simulink model "modelo_pink_noise"  (R2020a)
settings: Solver=ode15s  StartTime=0.0  StopTime=10  FixedStep=1/fs  MaxStep=1/(fs)  RelTol=1e-6
undefined symbols (not defined in the file): A, A_reduc, Amp, B, B_reduc, ba, Bdlol, C_reduc, Cc, D, den_anti, den_mems, dfilt, DiscIntNeverNeededParam, f0, fs, g, K_motor_virtual, ksi, ksia, L, Li, Lobs, n_adc, NSD_mems, num_anti, num_mems, obs_i_den, obs_i_num, obs_x2_den, obs_x2_num, R, R_control, sens_mems, v0, V_max, Vcc, Vmax_ADC, Vmin_ADC, x0
libraries: simulink x1, dspstat3 x1, dsparch4 x1, simulink_extras x1
settings Model: Creator=Noxi-PC  LastModifiedBy=Noxi-PC
settings SolverCC: ZeroCrossAlgorithm=Adaptive
settings DebuggingCC: IgnoredZcDiagnostic=none

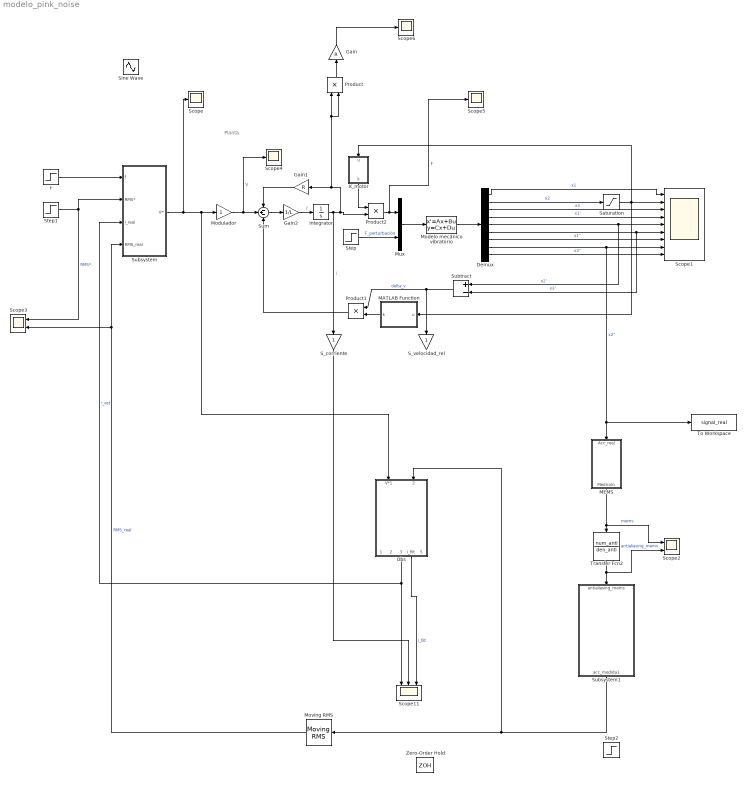
== system modelo_pink_noise ==
  note: Planta
  Demux : Demux  Outputs=9
  Gain : Gain  Gain=R
  Gain1 : Gain  Gain=R
  Gain2 : Gain  Gain=1/L
  Integrator : Integrator
  K_motor : MATLAB Function  TreatAsAtomicUnit=on
  MATLAB Function : MATLAB Function  TreatAsAtomicUnit=on
  MEMS : Subsystem
  Modelo mecánico vibratorio : StateSpace  A=A  B=B  C=Cc  D=D  InitialCondition=[x0,v0]
  Modulador : Gain
  Moving RMS : dspstat3/Moving RMS  Method=Sliding window  ForgettingFactorPort=off  SpecifyWindowLength=on  WindowLength=Ventana  ForgettingFactor=0.99  SimulateUsing=Interpreted execution
      settings: SourceProductBaseCode=DS
  Mux : Mux  Inputs=2
  Obs : Subsystem
  Product : Product
  Product1 : Product
  Product2 : Product
  S_corriente : Gain
  S_velocidad_rel : Gain
  Saturation : Saturate  UpperLimit=12.7e-3  LowerLimit=-12.7e-3
  Scope{,4..6} (4 alike) : Scope
  Scope1 : Scope  NumInputPorts=9
  Scope11 : Scope  NumInputPorts=3
  Scope2 : Scope  NumInputPorts=2
  Scope3 : Scope  NumInputPorts=2
  Sine Wave : Sin  Amplitude=5  Frequency=2*pi*f0  SampleTime=0
  Step : Step  After=0  SampleTime=0
  Step1 : Step  Time=0  After=Amp/sqrt(2)  SampleTime=0
  Step2 : Step  SampleTime=0
  Subsystem : Subsystem
  Subsystem1 : Subsystem
  Subtract : Sum  Inputs=+-
  Sum : Sum  Inputs=-+-
  To Workspace : ToWorkspace  VariableName=signal_real  SaveFormat=Structure With Time  SampleTime=-1
  Transfer Fcn2 : TransferFcn  Numerator=num_anti  Denominator=den_anti
  Zero-Order Hold : ZeroOrderHold  SampleTime=1/fs
  f : Step  Time=0  After=f0  SampleTime=0
  wires:
  Modelo mecánico vibratorio/1 -> Demux/1
  Demux/1 -> Scope1/1  "x1"
  Demux/2 -> Saturation/1  "x2"
  Demux/3 -> Scope1/3  "x3"
  Demux/4 -> Scope1/4  "x1'"
  Demux/5 -> Scope1/5, Subtract/1  "x2'"
  Demux/6 -> Scope1/6, Subtract/2  "x3'"
  Demux/7 -> Scope1/7  "x1''"
  Demux/8 -> To Workspace/1, MEMS/1(Acc_real), Scope1/8  "x2''"
  Demux/9 -> Scope1/9  "x3''"
  Mux/1 -> Modelo mecánico vibratorio/1
  Sum/1 -> Gain2/1
  Integrator/1 -> S_corriente/1, Product2/2, Gain1/1, Product/2, Product/1  "i"
  Gain1/1 -> Sum/1
  Gain2/1 -> Integrator/1  "i'"
  Step/1 -> Mux/2  "F_perturbación"
  Product1/1 -> Sum/3
  Subtract/1 -> Product1/1, S_velocidad_rel/1  "delta_v"
  Modulador/1 -> Scope4/1, Sum/2  "V"
  Saturation/1 -> K_motor/1(u), MATLAB Function/1(u), Scope1/2
  Product2/1 -> Scope5/1, Mux/1  "F"
  K_motor/1(k) -> Product2/1
  MATLAB Function/1(k) -> Product1/2
  f/1 -> Subsystem/1(f)
  Step1/1 -> Subsystem/2(RMS*), Scope3/1  "RMS*"
  Subsystem/1(V*') -> Scope/1, Obs/1(V*1), Modulador/1
  MEMS/1(Medición) -> Scope2/1, Transfer Fcn2/1  "mems"
  Obs/3(i_est) -> Subsystem/3(i_real), Scope11/1  "i_est"
  Obs/4(i_filt) -> Scope11/3  "i_filt"
  Moving RMS/1 -> Subsystem/4(RMS_real), Scope3/2  "RMS_real"
  Transfer Fcn2/1 -> Scope2/2, Subsystem1/1(antialiasing_mems)  "antialiasing_mems"
  S_corriente/1 -> Scope11/2
  Subsystem1/1(acc_medida1) -> Obs/2(acc_medida1), Moving RMS/1
  Product/1 -> Gain/1
  Gain/1 -> Scope6/1

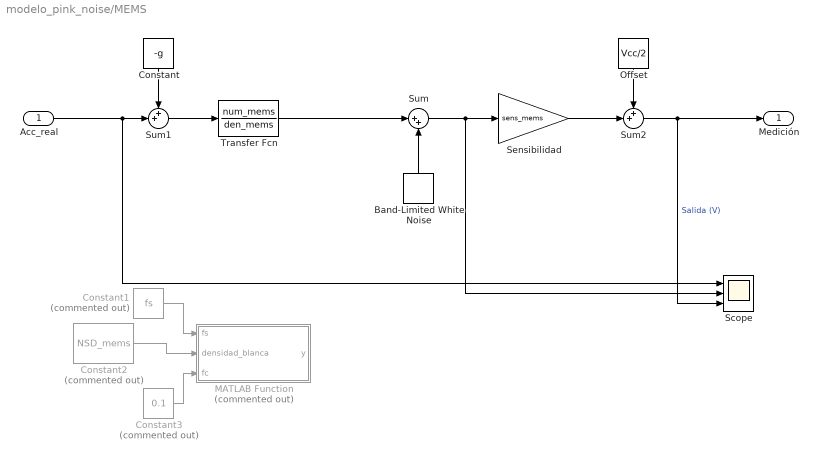
== system modelo_pink_noise/MEMS ==
  Acc_real : Inport
  Band-Limited White Noise : simulink/Sources/Band-Limited White Noise  Cov=NoisePower_mems  Ts=1/fs  seed=[23341]
  Constant : Constant  Value=-g
  Constant1 : Constant  Commented=on  Value=fs
  Constant2 : Constant  Commented=on  Value=NSD_mems
  Constant3 : Constant  Commented=on  Value=0.1
  MATLAB Function : MATLAB Function  Commented=on  TreatAsAtomicUnit=on
  Offset : Constant  Value=Vcc/2
  Scope : Scope  NumInputPorts=3
  Sensibilidad : Gain  Gain=sens_mems
  Sum : Sum  Inputs=|++
  Sum1 : Sum  Inputs=++|
  Sum2 : Sum  Inputs=++|
  Transfer Fcn : TransferFcn  Numerator=num_mems  Denominator=den_mems
  Medición : Outport
  wires:
  Sum1/1 -> Transfer Fcn/1
  Acc_real/1 -> Scope/1, Sum1/2
  Sum/1 -> Scope/2, Sensibilidad/1
  Sensibilidad/1 -> Sum2/2
  Sum2/1 -> Scope/3, Medición/1  "Salida (V)"
  Constant/1 -> Sum1/1
  Offset/1 -> Sum2/1
  Constant1/1 -> MATLAB Function/1(fs)
  Constant2/1 -> MATLAB Function/2(densidad_blanca)
  Constant3/1 -> MATLAB Function/3(fc)
  Transfer Fcn/1 -> Sum/1
  Band-Limited White Noise/1 -> Sum/2

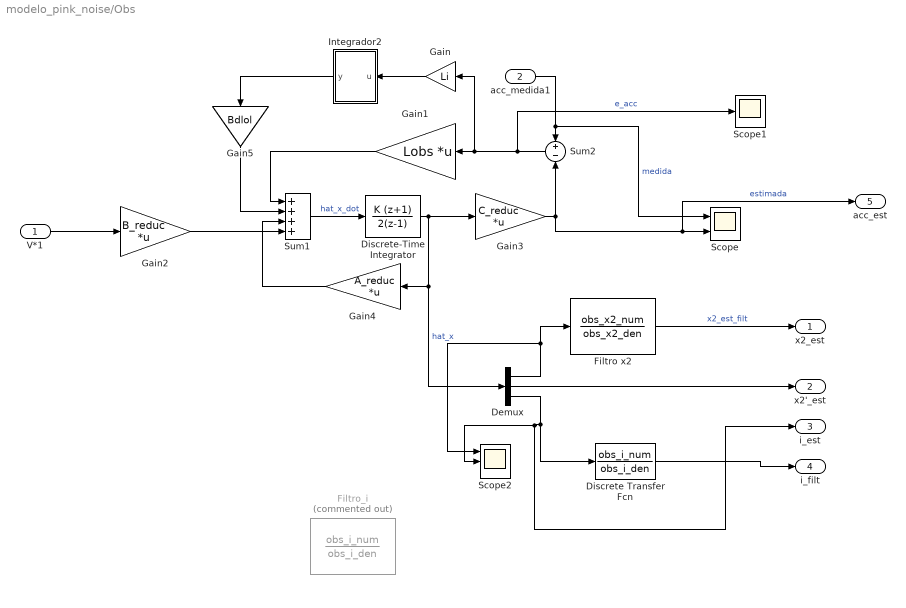
== system modelo_pink_noise/Obs ==
  V*1 : Inport
  acc_medida1 : Inport  Port=2
  Demux : Demux  Outputs=3
  Discrete Transfer Fcn : DiscreteTransferFcn  Numerator=obs_i_num  Denominator=obs_i_den  SampleTime=1/fs
  Discrete-Time Integrator : DiscreteIntegrator  IntegratorMethod=Accumulation: Trapezoidal  SampleTime=1/fs  ICPrevOutput=DiscIntNeverNeededParam  ICPrevScaledInput=DiscIntNeverNeededParam
  Filtro x2 : TransferFcn  Numerator=obs_x2_num  Denominator=obs_x2_den
  Filtro_i : TransferFcn  Commented=on  Numerator=obs_i_num  Denominator=obs_i_den
  Gain : Gain  Gain=Li
  Gain1 : Gain  Gain=Lobs  Multiplication=Matrix(K*u)
  Gain2 : Gain  Gain=B_reduc  Multiplication=Matrix(K*u)
  Gain3 : Gain  Gain=C_reduc  Multiplication=Matrix(K*u)
  Gain4 : Gain  Gain=A_reduc  Multiplication=Matrix(K*u)
  Gain5 : Gain  Gain=Bdlol
  Integrador2 : Subsystem
  Scope : Scope  NumInputPorts=2
  Scope1 : Scope
  Scope2 : Scope  NumInputPorts=3
  Sum1 : Sum  Inputs=++++
  Sum2 : Sum  Inputs=+|-
  x2_est : Outport
  x2'_est : Outport  Port=2
  i_est : Outport  Port=3
  i_filt : Outport  Port=4
  acc_est : Outport  Port=5
  wires:
  Gain1/1 -> Sum1/1
  Gain4/1 -> Sum1/3
  V*1/1 -> Gain2/1
  Sum2/1 -> Scope1/1, Gain/1, Gain1/1  "e_acc"
  Discrete-Time Integrator/1 -> Demux/1, Gain4/1, Gain3/1  "hat_x"
  Sum1/1 -> Discrete-Time Integrator/1  "hat_x_dot"
  acc_medida1/1 -> Scope/1, Sum2/1  "medida"
  Gain3/1 -> Sum2/2, acc_est/1, Scope/2  "estimada"
  Gain/1 -> Integrador2/1(u)
  Integrador2/1(y) -> Gain5/1
  Gain2/1 -> Sum1/4
  Demux/1 -> Scope2/1, Filtro x2/1
  Filtro x2/1 -> x2_est/1  "x2_est_filt"
  Demux/2 -> x2'_est/1
  Demux/3 -> Discrete Transfer Fcn/1, i_est/1, Scope2/2
  Discrete Transfer Fcn/1 -> i_filt/1
  Gain5/1 -> Sum1/2

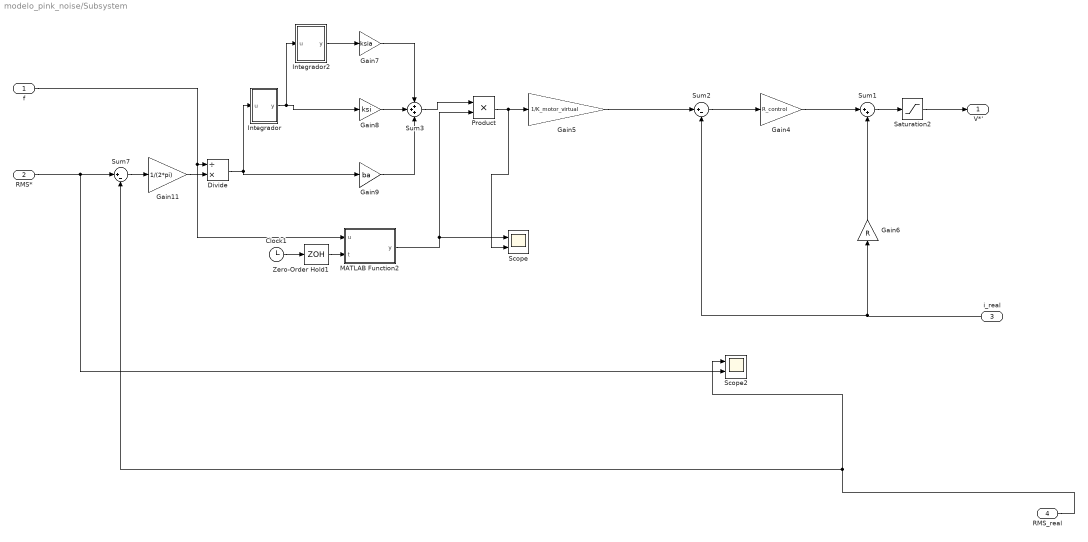
== system modelo_pink_noise/Subsystem ==
  f : Inport
  RMS* : Inport  Port=2
  i_real : Inport  Port=3
  RMS_real : Inport  Port=4
  Clock1 : Clock
  Divide : Product  Inputs=/*
  Gain11 : Gain  Gain=1/(2*pi)
  Gain4 : Gain  Gain=R_control
  Gain5 : Gain  Gain=1/K_motor_virtual
  Gain6 : Gain  Gain=R
  Gain7 : Gain  Gain=ksia
  Gain8 : Gain  Gain=ksi
  Gain9 : Gain  Gain=ba
  Integrador : Subsystem
  Integrador2 : Subsystem
  MATLAB Function2 : MATLAB Function  TreatAsAtomicUnit=on
  Product : Product
  Saturation2 : Saturate  UpperLimit=V_max  LowerLimit=-V_max
  Scope : Scope  NumInputPorts=2
  Scope2 : Scope  NumInputPorts=2
  Sum1 : Sum  Inputs=|++
  Sum2 : Sum  Inputs=|+-
  Sum3 : Sum  Inputs=+++
  Sum7 : Sum  Inputs=|+-
  Zero-Order Hold1 : ZeroOrderHold  SampleTime=1/fs
  V*' : Outport
  wires:
  Integrador2/1(y) -> Gain7/1
  Integrador/1(y) -> Gain8/1, Integrador2/1(u)
  RMS_real/1 -> Scope2/1, Sum7/2
  RMS*/1 -> Scope2/2, Sum7/1
  Gain8/1 -> Sum3/2
  Gain4/1 -> Sum1/1
  Sum2/1 -> Gain4/1
  Gain9/1 -> Sum3/3
  Sum7/1 -> Gain11/1
  i_real/1 -> Gain6/1, Sum2/2
  f/1 -> MATLAB Function2/1(u), Divide/1
  Gain6/1 -> Sum1/2
  Sum3/1 -> Product/1
  Product/1 -> Scope/2, Gain5/1
  Gain5/1 -> Sum2/1
  Gain11/1 -> Divide/2
  Gain7/1 -> Sum3/1
  Divide/1 -> Integrador/1(u), Gain9/1
  MATLAB Function2/1(y) -> Product/2, Scope/1
  Sum1/1 -> Saturation2/1
  Clock1/1 -> Zero-Order Hold1/1
  Zero-Order Hold1/1 -> MATLAB Function2/2(t)
  Saturation2/1 -> V*'/1

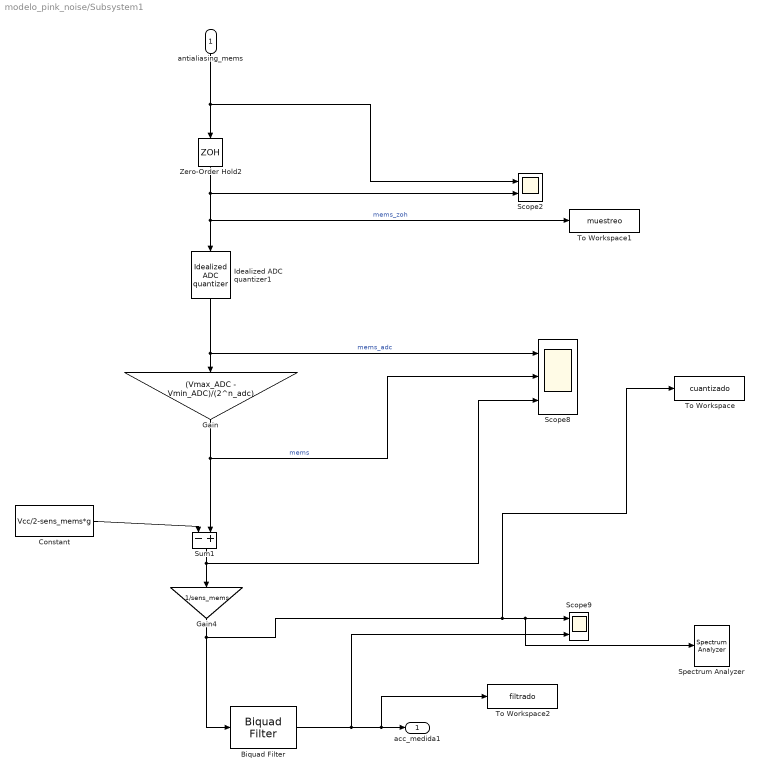
== system modelo_pink_noise/Subsystem1 ==
  antialiasing_mems : Inport
  Biquad Filter : dsparch4/Biquad Filter  FilterSource=Dialog parameters  CoeffSource=Specify via dialog  FilterObject=dfilt.df2tsos([1 0.3 0.4],[1 0.1 0.2])  IIRFiltStruct=Direct form II  BiQuadCoeffs=sos  ScaleValues=scaleV  IC=0  ICnum=0  ICden=0  a0Flag=Warning  optimizeScaleValues=on  ScaleValueMode=Specify via input port (g)  roundingMode=Floor  overflowMode=off  scaleValueFracLength=14  denProdOutputFracLength=30  denAccumFracLength=30  secondMemoryFracLength=15
  Constant : Constant  Value=Vcc/2-sens_mems*g
  Gain : Gain  Gain=(Vmax_ADC - Vmin_ADC)/(2^n_adc)
  Gain4 : Gain  Gain=1/sens_mems
  Idealized ADC quantizer1 : simulink_extras/Additional Discrete/Idealized ADC quantizer  NumberOfConverterBits=n_adc  Vmin=Vmin_ADC  Vmax=Vmax_ADC  OutputDataType=uint16  OutputNegativeValues=off
  Scope2 : Scope  NumInputPorts=2
  Scope8 : Scope  NumInputPorts=3
  Scope9 : Scope  NumInputPorts=2
  Spectrum Analyzer : SpectrumAnalyzer
  Sum1 : Sum  Inputs=-+
  To Workspace : ToWorkspace  VariableName=cuantizado  SaveFormat=Structure With Time  SampleTime=1/fs
  To Workspace1 : ToWorkspace  VariableName=muestreo  SaveFormat=Structure With Time  SampleTime=1/fs
  To Workspace2 : ToWorkspace  VariableName=filtrado  SaveFormat=Structure With Time  SampleTime=1/fs
  Zero-Order Hold2 : ZeroOrderHold  SampleTime=1/(fs)
  acc_medida1 : Outport
  wires:
  Gain4/1 -> Biquad Filter/1, To Workspace/1, Spectrum Analyzer/1, Scope9/1
  Gain/1 -> Scope8/2, Sum1/2  "mems"
  Idealized ADC quantizer1/1 -> Gain/1, Scope8/1  "mems_adc"
  Sum1/1 -> Scope8/3, Gain4/1
  antialiasing_mems/1 -> Scope2/1, Zero-Order Hold2/1
  Zero-Order Hold2/1 -> To Workspace1/1, Idealized ADC quantizer1/1, Scope2/2  "mems_zoh"
  Biquad Filter/1 -> Scope9/2, To Workspace2/1, acc_medida1/1
  Constant/1 -> Sum1/1

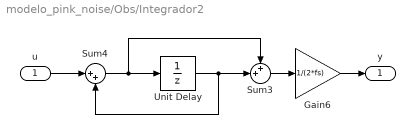
== system modelo_pink_noise/Obs/Integrador2 ==
  u : Inport
  Gain6 : Gain  Gain=1/(2*fs)
  Sum3 : Sum  Inputs=++|
  Sum4 : Sum  Inputs=|++
  Unit Delay : UnitDelay  SampleTime=1/fs  HasFrameUpgradeWarning=on
  y : Outport
  wires:
  Sum3/1 -> Gain6/1
  Sum4/1 -> Sum3/1, Unit Delay/1
  Unit Delay/1 -> Sum3/2, Sum4/2
  Gain6/1 -> y/1
  u/1 -> Sum4/1

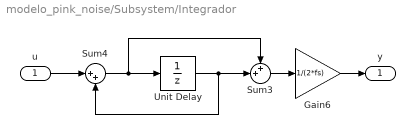
== system modelo_pink_noise/Subsystem/Integrador ==
  u : Inport
  Gain6 : Gain  Gain=1/(2*fs)
  Sum3 : Sum  Inputs=++|
  Sum4 : Sum  Inputs=|++
  Unit Delay : UnitDelay  SampleTime=1/fs  HasFrameUpgradeWarning=on
  y : Outport
  wires:
  Sum3/1 -> Gain6/1
  Sum4/1 -> Sum3/1, Unit Delay/1
  Unit Delay/1 -> Sum3/2, Sum4/2
  Gain6/1 -> y/1
  u/1 -> Sum4/1

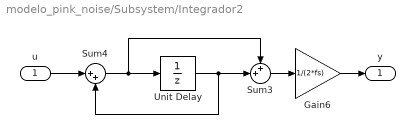
== system modelo_pink_noise/Subsystem/Integrador2 ==
  u : Inport
  Gain6 : Gain  Gain=1/(2*fs)
  Sum3 : Sum  Inputs=++|
  Sum4 : Sum  Inputs=|++
  Unit Delay : UnitDelay  SampleTime=1/fs  HasFrameUpgradeWarning=on
  y : Outport
  wires:
  Sum3/1 -> Gain6/1
  Sum4/1 -> Sum3/1, Unit Delay/1
  Unit Delay/1 -> Sum3/2, Sum4/2
  Gain6/1 -> y/1
  u/1 -> Sum4/1

== matlab function modelo_pink_noise/MATLAB Function ==
  data: u input; k output
function k= fcn(u)
coefs = [1883883250149.81,121220914.941173,-604988778.285297,-369001.905871325,-43371.4523559472,-47.4444922489166,51.4222931299995];

k = coefs(1)*u^6+coefs(2)*u^5+coefs(3)*u^4+coefs(4)*u^3+coefs(5)*u^2+coefs(6)*u^1+coefs(7);

== matlab function modelo_pink_noise/MEMS/MATLAB Function ==
  data: fs input; y output; densidad_blanca input; fc input
function y = ruido_sensor(fs, densidad_blanca, fc)

% Persistent state
persistent b a z

if isempty(b)
    [b, a] = butter(1, fc/(fs/2));
    z = 0;  % Estado inicial del filtro
end

% Ruido blanco
ruido_blanco = densidad_blanca * randn * sqrt(fs);

% Ruido 1/f (drift)
[ruido_drift, z] = filter(b, a, randn, z);

% Señal total
y = ruido_blanco + ruido_drift;

== matlab function modelo_pink_noise/Subsystem/MATLAB Function2 ==
  data: u input; y output; t input
function y = fcn(u,t)

y = sin(2*pi*u*t);

== matlab function modelo_pink_noise/K_motor ==
  data: u input; k output
function k = fcn(u)
coefs = [1.88388325014986e-06,1.21220914940963e-07,-0.000604988778285308,-0.000369001905871298,-0.0433714523559467,-0.0474444922489168,51.4222931299995];

k = coefs(1)*u^6+coefs(2)*u^5+coefs(3)*u^4+coefs(4)*u^3+coefs(5)*u^2+coefs(6)*u^1+coefs(7);
